simulink model "bee2_complex_corr"  (Simulink 7.0)
settings: Solver=ode45  StartTime=0.0  StopTime=10.0  RelTol=1e-3
undefined symbols (not defined in the file or in its folder): BEE2_usr
libraries: xbsIndex_r4 x279, xps_library x61, casper_library_misc x18
(part 3 of 4)

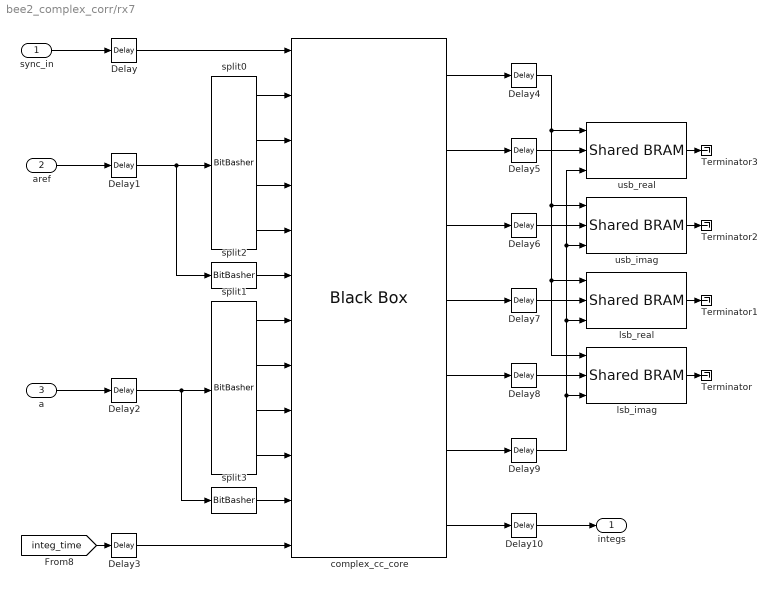
== system bee2_complex_corr/rx7 ==
  sync_in : Inport  OutDataType=sfix(16)  OutScaling=2^0
  aref : Inport  Port=2  OutDataType=sfix(16)  OutScaling=2^0
  a : Inport  Port=3  OutDataType=sfix(16)  OutScaling=2^0
  Delay{,1..10} (11 alike) : xbsIndex_r4/Delay  en=off  latency=1  dbl_ovrd=off  reg_retiming=off  block_type=delay
  Terminator{,1..3} (4 alike) : Terminator
  complex_cc_core : xbsIndex_r4/Black Box  init_code=complex_cc_core_config  sim_method=Inactive  block_type=blackbox2
      settings: infoedit="Incorporates black box HDL and simulation model into a System Generator design.<P><P>You must supply a Black Box with certain information about the HDL component you would like to bring into System Generator. This information is provided through a Matlab function.<P><P>When \"Simulation mode\" is set to \"Inactive\", you will typically want to provide a separate simulation model by using a Simulation Multiplexer.<P>When \"Simulation mode\" is set to \"External co-simulator\", you must include a ModelSim block in the design."  block_version=10.1.3
  lsb_imag : xps_library/Shared BRAM  Tag=xps:bram  SystemSampleTime=-1  arith_type="Signed  (2's comp)"  addr_width=11  data_width=32  data_bin_pt=0  init_vals=0  sample_rate=1
      link override bee2_complex_corr_0x0_func_real_data_out: arith_type="Signed  (2's comp)"
      link override bee2_complex_corr_corr00_func_real_data_out: arith_type="Signed  (2's comp)"
      link override bee2_complex_corr_corr01_func_real_data_out: arith_type="Signed  (2's comp)"
      link override bee2_complex_corr_rx7_lsb_imag_data_out: arith_type="Signed  (2's comp)"
      link override convert_din: arith_type="Signed  (2's comp)"
      link override correlator_2bit_bee2_output_corr0_data_out: arith_type=Unsigned
      link override correlator_2bit_bee2_x2_output_corr01_data_out: arith_type=Unsigned
      link override correlator_2bit_bee2_x2_output_corr0_data_out: arith_type=Unsigned
      link override correlator_2bit_ibob_output_corr0_data_out: arith_type=Unsigned
      link override cross_correlator_test_corr_out_data_out: arith_type="Signed  (2's comp)"
      link override cross_correlator_test_input_data1_data_out: arith_type=Unsigned
      link override dbe_xaui_corr_corr_func_data_out: arith_type="Signed  (2's comp)"
      link override dbe_xaui_corr_new_xaui_summer_summer_output_corr_data_out: arith_type="Signed  (2's comp)"
      link override dbe_xaui_corr_xaui_summer_summer_output_corr_data_out: arith_type="Signed  (2's comp)"
      link override mem/sim_data_in: arith_type="Signed  (2's comp)"
  lsb_real : xps_library/Shared BRAM  Tag=xps:bram  SystemSampleTime=-1  arith_type="Signed  (2's comp)"  addr_width=11  data_width=32  data_bin_pt=0  init_vals=0  sample_rate=1
      link override bee2_complex_corr_0x0_func_real_data_out: arith_type="Signed  (2's comp)"
      link override bee2_complex_corr_corr00_func_real_data_out: arith_type="Signed  (2's comp)"
      link override bee2_complex_corr_corr01_func_real_data_out: arith_type="Signed  (2's comp)"
      link override bee2_complex_corr_rx7_lsb_real_data_out: arith_type="Signed  (2's comp)"
      link override convert_din: arith_type="Signed  (2's comp)"
      link override correlator_2bit_bee2_output_corr0_data_out: arith_type=Unsigned
      link override correlator_2bit_bee2_x2_output_corr01_data_out: arith_type=Unsigned
      link override correlator_2bit_bee2_x2_output_corr0_data_out: arith_type=Unsigned
      link override correlator_2bit_ibob_output_corr0_data_out: arith_type=Unsigned
      link override cross_correlator_test_corr_out_data_out: arith_type="Signed  (2's comp)"
      link override cross_correlator_test_input_data1_data_out: arith_type=Unsigned
      link override dbe_xaui_corr_corr_func_data_out: arith_type="Signed  (2's comp)"
      link override dbe_xaui_corr_new_xaui_summer_summer_output_corr_data_out: arith_type="Signed  (2's comp)"
      link override dbe_xaui_corr_xaui_summer_summer_output_corr_data_out: arith_type="Signed  (2's comp)"
      link override mem/sim_data_in: arith_type="Signed  (2's comp)"
  split0 : xbsIndex_r4/BitBasher  bitexpr=|  display_expr=off  sr_1=1  arith_type1=Unsigned  bin_pt1=0  sr_2=2  arith_type2=Unsigned  bin_pt2=0  sr_3=3  arith_type3=Unsigned  bin_pt3=0  sr_4=4  arith_type4=Unsigned  bin_pt4=0  dbl_ovrd=off  block_type=bitbasher
      | <html><head><meta name="qrichtext" content="1" /><style type="text/css">
      | p, li { white-space: pre-wrap; }
      | </style></head><body style=" font-family:'MS Shell Dlg 2'; font-size:8.25pt; font-weight:400; font-style:normal;">
      | <p style=" margin-top:0px; margin-bottom:0px; margin-left:0px; margin-right:0px; -qt-block-indent:0; text-indent:0px; font-size:8pt;">r0={a[8:7]}<br />i0={a[6:5]}<br /><span style=" font-family:'MS Shell Dlg';">r1={a[4:3]}<br />i1={a[2:1]}</span></p></body></html>
      settings: block_version=10.1.3
  split1 : xbsIndex_r4/BitBasher  bitexpr=|  display_expr=off  sr_1=1  arith_type1=Unsigned  bin_pt1=0  sr_2=2  arith_type2=Unsigned  bin_pt2=0  sr_3=3  arith_type3=Unsigned  bin_pt3=0  sr_4=4  arith_type4=Unsigned  bin_pt4=0  dbl_ovrd=off  block_type=bitbasher
      | <html><head><meta name="qrichtext" content="1" /><style type="text/css">
      | p, li { white-space: pre-wrap; }
      | </style></head><body style=" font-family:'MS Shell Dlg 2'; font-size:8.25pt; font-weight:400; font-style:normal;">
      | <p style=" margin-top:0px; margin-bottom:0px; margin-left:0px; margin-right:0px; -qt-block-indent:0; text-indent:0px; font-size:8pt;">r0={a[8:7]}<br />i0={a[6:5]}<br /><span style=" font-family:'MS Shell Dlg';">r1={a[4:3]}<br />i1={a[2:1]}</span></p></body></html>
      settings: block_version=10.1.3
  split2 : xbsIndex_r4/BitBasher  bitexpr=|  display_expr=off  sr_1=1  arith_type1=Unsigned  bin_pt1=0  sr_2=2  arith_type2=Unsigned  bin_pt2=0  sr_3=3  arith_type3=Unsigned  bin_pt3=0  sr_4=4  arith_type4=Unsigned  bin_pt4=0  dbl_ovrd=off  block_type=bitbasher
      | <html><head><meta name="qrichtext" content="1" /><style type="text/css">
      | p, li { white-space: pre-wrap; }
      | </style></head><body style=" font-family:'MS Shell Dlg 2'; font-size:8.25pt; font-weight:400; font-style:normal;">
      | <p style=" margin-top:0px; margin-bottom:0px; margin-left:0px; margin-right:0px; -qt-block-indent:0; text-indent:0px; font-size:8pt;"><span style=" font-family:'MS Shell Dlg';">w={a[0]}</span></p></body></html>
      settings: block_version=10.1.3
  split3 : xbsIndex_r4/BitBasher  bitexpr=|  display_expr=off  sr_1=1  arith_type1=Unsigned  bin_pt1=0  sr_2=2  arith_type2=Unsigned  bin_pt2=0  sr_3=3  arith_type3=Unsigned  bin_pt3=0  sr_4=4  arith_type4=Unsigned  bin_pt4=0  dbl_ovrd=off  block_type=bitbasher
      | <html><head><meta name="qrichtext" content="1" /><style type="text/css">
      | p, li { white-space: pre-wrap; }
      | </style></head><body style=" font-family:'MS Shell Dlg 2'; font-size:8.25pt; font-weight:400; font-style:normal;">
      | <p style=" margin-top:0px; margin-bottom:0px; margin-left:0px; margin-right:0px; -qt-block-indent:0; text-indent:0px; font-size:8pt;"><span style=" font-family:'MS Shell Dlg';">w={a[0]}</span></p></body></html>
      settings: block_version=10.1.3
  usb_imag : xps_library/Shared BRAM  Tag=xps:bram  SystemSampleTime=-1  arith_type="Signed  (2's comp)"  addr_width=11  data_width=32  data_bin_pt=0  init_vals=0  sample_rate=1
      link override bee2_complex_corr_0x0_func_real_data_out: arith_type="Signed  (2's comp)"
      link override bee2_complex_corr_corr00_func_real_data_out: arith_type="Signed  (2's comp)"
      link override bee2_complex_corr_corr01_func_real_data_out: arith_type="Signed  (2's comp)"
      link override bee2_complex_corr_rx7_usb_imag_data_out: arith_type="Signed  (2's comp)"
      link override convert_din: arith_type="Signed  (2's comp)"
      link override correlator_2bit_bee2_output_corr0_data_out: arith_type=Unsigned
      link override correlator_2bit_bee2_x2_output_corr01_data_out: arith_type=Unsigned
      link override correlator_2bit_bee2_x2_output_corr0_data_out: arith_type=Unsigned
      link override correlator_2bit_ibob_output_corr0_data_out: arith_type=Unsigned
      link override cross_correlator_test_corr_out_data_out: arith_type="Signed  (2's comp)"
      link override cross_correlator_test_input_data1_data_out: arith_type=Unsigned
      link override dbe_xaui_corr_corr_func_data_out: arith_type="Signed  (2's comp)"
      link override dbe_xaui_corr_new_xaui_summer_summer_output_corr_data_out: arith_type="Signed  (2's comp)"
      link override dbe_xaui_corr_xaui_summer_summer_output_corr_data_out: arith_type="Signed  (2's comp)"
      link override mem/sim_data_in: arith_type="Signed  (2's comp)"
  usb_real : xps_library/Shared BRAM  Tag=xps:bram  SystemSampleTime=-1  arith_type="Signed  (2's comp)"  addr_width=11  data_width=32  data_bin_pt=0  init_vals=0  sample_rate=1
      link override bee2_complex_corr_0x0_func_real_data_out: arith_type="Signed  (2's comp)"
      link override bee2_complex_corr_corr00_func_real_data_out: arith_type="Signed  (2's comp)"
      link override bee2_complex_corr_corr01_func_real_data_out: arith_type="Signed  (2's comp)"
      link override bee2_complex_corr_rx7_usb_real_data_out: arith_type="Signed  (2's comp)"
      link override convert_din: arith_type="Signed  (2's comp)"
      link override correlator_2bit_bee2_output_corr0_data_out: arith_type=Unsigned
      link override correlator_2bit_bee2_x2_output_corr01_data_out: arith_type=Unsigned
      link override correlator_2bit_bee2_x2_output_corr0_data_out: arith_type=Unsigned
      link override correlator_2bit_ibob_output_corr0_data_out: arith_type=Unsigned
      link override cross_correlator_test_corr_out_data_out: arith_type="Signed  (2's comp)"
      link override cross_correlator_test_input_data1_data_out: arith_type=Unsigned
      link override dbe_xaui_corr_corr_func_data_out: arith_type="Signed  (2's comp)"
      link override dbe_xaui_corr_new_xaui_summer_summer_output_corr_data_out: arith_type="Signed  (2's comp)"
      link override dbe_xaui_corr_xaui_summer_summer_output_corr_data_out: arith_type="Signed  (2's comp)"
      link override mem/sim_data_in: arith_type="Signed  (2's comp)"
  integs : Outport  OutDataType=sfix(16)  OutScaling=2^0
  wires:
  [integ_time] -> Delay3/1
  a/1 -> Delay2/1
  aref/1 -> Delay1/1
  split0/4 -> complex_cc_core/5
  split0/3 -> complex_cc_core/4
  split0/2 -> complex_cc_core/3
  split0/1 -> complex_cc_core/2
  sync_in/1 -> Delay/1
  complex_cc_core/1 -> Delay4/1
  complex_cc_core/2 -> Delay5/1
  complex_cc_core/3 -> Delay6/1
  complex_cc_core/4 -> Delay7/1
  complex_cc_core/5 -> Delay8/1
  Delay/1 -> complex_cc_core/1
  Delay1/1 -> split0/1, split2/1
  Delay2/1 -> split1/1, split3/1
  Delay7/1 -> lsb_real/2
  Delay8/1 -> lsb_imag/2
  Delay10/1 -> integs/1
  complex_cc_core/6 -> Delay9/1
  complex_cc_core/7 -> Delay10/1
  Delay5/1 -> usb_real/2
  Delay6/1 -> usb_imag/2
  Delay3/1 -> complex_cc_core/12
  split2/1 -> complex_cc_core/6
  split1/1 -> complex_cc_core/7
  split1/2 -> complex_cc_core/8
  split1/3 -> complex_cc_core/9
  split1/4 -> complex_cc_core/10
  split3/1 -> complex_cc_core/11
  Delay4/1 -> usb_real/1, usb_imag/1, lsb_imag/1, lsb_real/1
  Delay9/1 -> usb_real/3, usb_imag/3, lsb_real/3, lsb_imag/3
  lsb_imag/1 -> Terminator/1
  lsb_real/1 -> Terminator1/1
  usb_imag/1 -> Terminator2/1
  usb_real/1 -> Terminator3/1

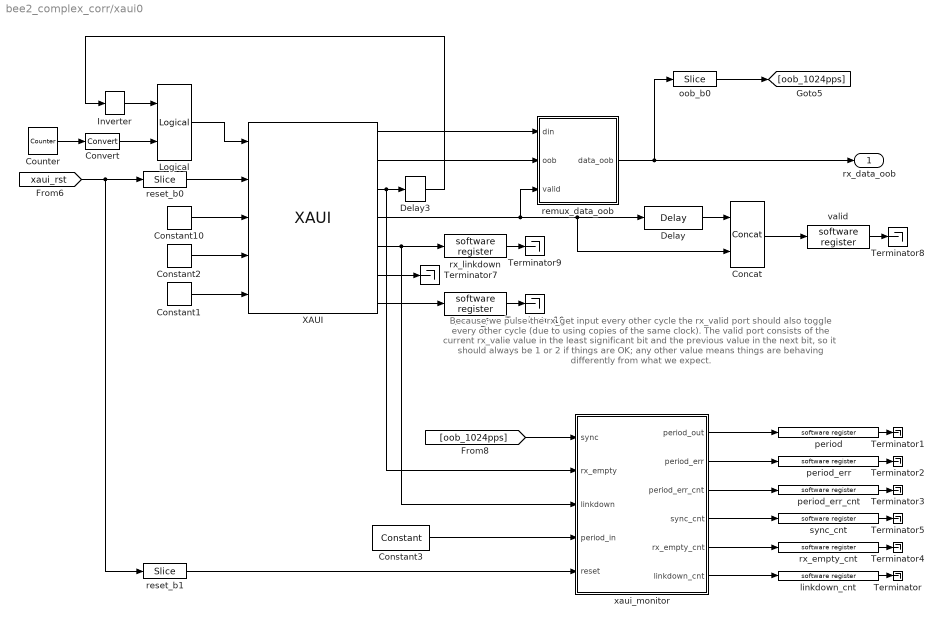
== system bee2_complex_corr/xaui0 ==
  note: Because we pulse the rx_get input every other cycle
      | the rx_valid port should also toggle every other cycle
      | (due to using copies of the same clock).  The valid port
      | consists of the current rx_valie value in the least significant
      | bit and the previous value in the next bit, so it should
      | always be 1 or 2 if things are OK; any other value means
      | things are behaving differently from what we expect.
  Concat : xbsIndex_r4/Concat  num_inputs=2  dbl_ovrd=off  block_type=concat
      settings: block_version=10.1.3
  Constant1 : xbsIndex_r4/Constant  arith_type=Boolean  const=0  n_bits=4  bin_pt=0  explicit_period=on  period=1  equ=P=C  opselect=C  inp2=PCIN>>17  opr=+  inp1=P  carry=CIN  dbl_ovrd=off  block_type=constant
      settings: block_version=11.3
  Constant10 : xbsIndex_r4/Constant  arith_type=Unsigned  const=2^4 -1  n_bits=32  bin_pt=0  explicit_period=on  period=1  equ=P=C  opselect=C  inp2=PCIN>>17  opr=+  inp1=P  carry=CIN  dbl_ovrd=off  block_type=constant
      settings: block_version=11.3
  Constant2 : xbsIndex_r4/Constant  arith_type=Unsigned  const=0  n_bits=4  bin_pt=0  explicit_period=on  period=1  equ=P=C  opselect=C  inp2=PCIN>>17  opr=+  inp1=P  carry=CIN  dbl_ovrd=off  block_type=constant
      settings: block_version=11.3
  Constant3 : xbsIndex_r4/Constant  arith_type=Unsigned  const=1e6/4  n_bits=32  bin_pt=0  explicit_period=on  period=1  equ=P=C  opselect=C  inp2=PCIN>>17  opr=+  inp1=P  carry=CIN  dbl_ovrd=off  block_type=constant
      settings: block_version=11.3
  Convert : xbsIndex_r4/Convert  arith_type=Boolean  n_bits=16  bin_pt=14  quantization=Truncate  overflow=Wrap  latency=0  dbl_ovrd=off  pipeline=off  block_type=convert
      settings: block_version=10.1.3
  Counter : xbsIndex_r4/Counter  cnt_type=Free Running  cnt_to=Inf  operation=Up  start_count=0  cnt_by_val=1  arith_type=Unsigned  n_bits=1  bin_pt=0  load_pin=off  rst=off  en=off  explicit_period=on  period=1  dbl_ovrd=off  use_behavioral_HDL=off  use_rpm=off  implementation=Fabric  block_type=counter
  Delay : xbsIndex_r4/Delay  en=off  latency=1  dbl_ovrd=off  reg_retiming=off  block_type=delay
  Delay3 : xbsIndex_r4/Delay  en=off  latency=32  dbl_ovrd=off  reg_retiming=off  block_type=delay
      settings: block_version=11.3
  Inverter : xbsIndex_r4/Inverter  en=off  latency=0  dbl_ovrd=off  block_type=inv
      settings: block_version=11.3
  Logical : xbsIndex_r4/Logical  logical_function=AND  inputs=2  en=off  latency=0  precision=Full  arith_type=Unsigned  n_bits=16  bin_pt=0  align_bp=on  dbl_ovrd=off  block_type=logical
  Terminator{,1..5,7..10} (10 alike) : Terminator
  XAUI : xps_library/XAUI  Tag=xps:xaui  SystemSampleTime=-1  demux=1  port=BEE2_usr:0  open_phy=off  show_param=off  pre_emph=3  swing=800
      link override bee2_complex_corr_xaui0_XAUI_rx_data: n_bits=64
      link override bee2_complex_corr_xaui0_XAUI_rx_outofband: n_bits=8
      link override convert_tx_data: n_bits=64
      link override convert_tx_outofband: n_bits=8
      link override dbe_xaui_corr_xaui0_XAUI_rx_data: n_bits=64
      link override dbe_xaui_corr_xaui0_XAUI_rx_outofband: n_bits=8
      link override dbe_xaui_corr_xaui1_XAUI_rx_data: n_bits=64
      link override dbe_xaui_corr_xaui1_XAUI_rx_outofband: n_bits=8
      link override dbe_xaui_corr_xaui_summer_XAUI0_rx_data: n_bits=32
      link override dbe_xaui_corr_xaui_summer_XAUI0_rx_outofband: n_bits=4
      link override dbe_xaui_xaui_summer_XAUI0_rx_data: n_bits=32
      link override dbe_xaui_xaui_summer_XAUI0_rx_outofband: n_bits=4
      link override xaui_XAUI_RECV_rx_data: n_bits=32
      link override xaui_XAUI_RECV_rx_outofband: n_bits=4
  almost_full : xps_library/software register  Tag=xps:sw_reg  SystemSampleTime=-1  io_dir=To Processor  arith_type=Unsigned  bitwidth=32  bin_pt=0  sample_period=1  gw_name=bee2_complex_corr_xaui0_almost_full_user_data_in
      link override convert: arith_type=Unsigned  n_bits=32  bin_pt=0
  linkdown_cnt : xps_library/software register  Tag=xps:sw_reg  SystemSampleTime=-1  io_dir=To Processor  arith_type=Unsigned  bitwidth=32  bin_pt=0  sample_period=1  gw_name=bee2_complex_corr_xaui0_linkdown_cnt_user_data_in
      link override convert: arith_type=Unsigned  n_bits=32  bin_pt=0
  oob_b0 : xbsIndex_r4/Slice  nbits=1  boolean_output=on  mode=Lower Bit Location + Width  bit1=0  base1=MSB of Input  bit0=0  base0=LSB of Input  dbl_ovrd=off  block_type=slice
      settings: block_version=11.3
  period : xps_library/software register  Tag=xps:sw_reg  SystemSampleTime=-1  io_dir=To Processor  arith_type=Unsigned  bitwidth=32  bin_pt=0  sample_period=1  gw_name=bee2_complex_corr_xaui0_period_user_data_in
      link override convert: arith_type=Unsigned  n_bits=32  bin_pt=0
  period_err : xps_library/software register  Tag=xps:sw_reg  SystemSampleTime=-1  io_dir=To Processor  arith_type=Unsigned  bitwidth=32  bin_pt=0  sample_period=1  gw_name=bee2_complex_corr_xaui0_period_err_user_data_in
      link override convert: arith_type=Unsigned  n_bits=32  bin_pt=0
  period_err_cnt : xps_library/software register  Tag=xps:sw_reg  SystemSampleTime=-1  io_dir=To Processor  arith_type=Unsigned  bitwidth=32  bin_pt=0  sample_period=1  gw_name=bee2_complex_corr_xaui0_period_err_cnt_user_data_in
      link override convert: arith_type=Unsigned  n_bits=32  bin_pt=0
  remux_data_oob : Subsystem
  reset_b0 : xbsIndex_r4/Slice  nbits=1  boolean_output=on  mode=Lower Bit Location + Width  bit1=0  base1=MSB of Input  bit0=0  base0=LSB of Input  dbl_ovrd=off  block_type=slice
      settings: block_version=11.3
  reset_b1 : xbsIndex_r4/Slice  nbits=1  boolean_output=on  mode=Lower Bit Location + Width  bit1=0  base1=MSB of Input  bit0=1  base0=LSB of Input  dbl_ovrd=off  block_type=slice
      settings: block_version=11.3
  rx_empty_cnt : xps_library/software register  Tag=xps:sw_reg  SystemSampleTime=-1  io_dir=To Processor  arith_type=Unsigned  bitwidth=32  bin_pt=0  sample_period=1  gw_name=bee2_complex_corr_xaui0_rx_empty_cnt_user_data_in
      link override convert: arith_type=Unsigned  n_bits=32  bin_pt=0
  rx_linkdown : xps_library/software register  Tag=xps:sw_reg  SystemSampleTime=-1  io_dir=To Processor  arith_type=Unsigned  bitwidth=32  bin_pt=0  sample_period=1  gw_name=bee2_complex_corr_xaui0_rx_linkdown_user_data_in
      link override convert: arith_type=Unsigned  n_bits=32  bin_pt=0
  sync_cnt : xps_library/software register  Tag=xps:sw_reg  SystemSampleTime=-1  io_dir=To Processor  arith_type=Unsigned  bitwidth=32  bin_pt=0  sample_period=1  gw_name=bee2_complex_corr_xaui0_sync_cnt_user_data_in
      link override convert: arith_type=Unsigned  n_bits=32  bin_pt=0
  valid : xps_library/software register  Tag=xps:sw_reg  SystemSampleTime=-1  io_dir=To Processor  arith_type=Unsigned  bitwidth=32  bin_pt=0  sample_period=1  gw_name=bee2_complex_corr_xaui0_valid_user_data_in
      link override convert: arith_type=Unsigned  n_bits=32  bin_pt=0
  xaui_monitor : Subsystem
  rx_data_oob : Outport
  wires:
  Constant2/1 -> XAUI/4
  XAUI/3 -> Delay3/1, xaui_monitor/2(rx_empty)
  Delay3/1 -> Inverter/1
  XAUI/6 -> Terminator7/1
  Constant10/1 -> XAUI/3
  XAUI/4 -> Delay/1, Concat/2, remux_data_oob/3(valid)
  XAUI/5 -> rx_linkdown/1, xaui_monitor/3(linkdown)
  valid/1 -> Terminator8/1
  rx_linkdown/1 -> Terminator9/1
  almost_full/1 -> Terminator10/1
  XAUI/7 -> almost_full/1
  Constant1/1 -> XAUI/5
  [xaui_rst] -> reset_b0/1, reset_b1/1
  Inverter/1 -> Logical/1
  Logical/1 -> XAUI/1
  Counter/1 -> Convert/1
  XAUI/1 -> remux_data_oob/1(din)
  Concat/1 -> valid/1
  Delay/1 -> Concat/1
  Convert/1 -> Logical/2
  remux_data_oob/1(data_oob) -> oob_b0/1, rx_data_oob/1
  reset_b0/1 -> XAUI/2
  reset_b1/1 -> xaui_monitor/5(reset)
  Constant3/1 -> xaui_monitor/4(period_in)
  [oob_1024pps] -> xaui_monitor/1(sync)
  oob_b0/1 -> [oob_1024pps]
  xaui_monitor/1(period_out) -> period/1
  xaui_monitor/2(period_err) -> period_err/1
  xaui_monitor/3(period_err_cnt) -> period_err_cnt/1
  xaui_monitor/4(sync_cnt) -> sync_cnt/1
  xaui_monitor/5(rx_empty_cnt) -> rx_empty_cnt/1
  xaui_monitor/6(linkdown_cnt) -> linkdown_cnt/1
  linkdown_cnt/1 -> Terminator/1
  period/1 -> Terminator1/1
  period_err/1 -> Terminator2/1
  period_err_cnt/1 -> Terminator3/1
  rx_empty_cnt/1 -> Terminator4/1
  sync_cnt/1 -> Terminator5/1
  XAUI/2 -> remux_data_oob/2(oob)

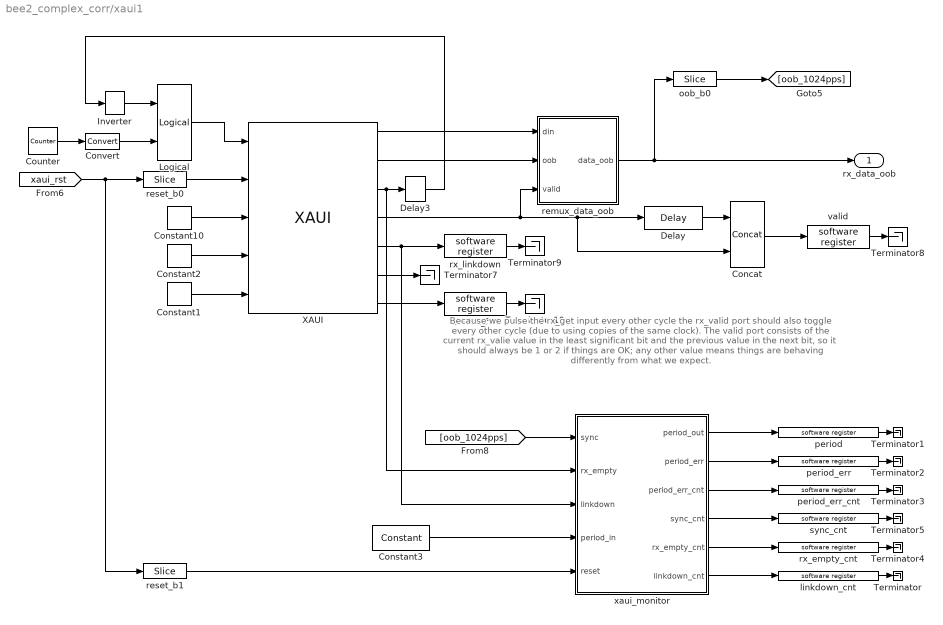
== system bee2_complex_corr/xaui1 ==
  note: Because we pulse the rx_get input every other cycle
      | the rx_valid port should also toggle every other cycle
      | (due to using copies of the same clock).  The valid port
      | consists of the current rx_valie value in the least significant
      | bit and the previous value in the next bit, so it should
      | always be 1 or 2 if things are OK; any other value means
      | things are behaving differently from what we expect.
  Concat : xbsIndex_r4/Concat  num_inputs=2  dbl_ovrd=off  block_type=concat
      settings: block_version=10.1.3
  Constant1 : xbsIndex_r4/Constant  arith_type=Boolean  const=0  n_bits=4  bin_pt=0  explicit_period=on  period=1  equ=P=C  opselect=C  inp2=PCIN>>17  opr=+  inp1=P  carry=CIN  dbl_ovrd=off  block_type=constant
      settings: block_version=11.3
  Constant10 : xbsIndex_r4/Constant  arith_type=Unsigned  const=2^4 -1  n_bits=32  bin_pt=0  explicit_period=on  period=1  equ=P=C  opselect=C  inp2=PCIN>>17  opr=+  inp1=P  carry=CIN  dbl_ovrd=off  block_type=constant
      settings: block_version=11.3
  Constant2 : xbsIndex_r4/Constant  arith_type=Unsigned  const=0  n_bits=4  bin_pt=0  explicit_period=on  period=1  equ=P=C  opselect=C  inp2=PCIN>>17  opr=+  inp1=P  carry=CIN  dbl_ovrd=off  block_type=constant
      settings: block_version=11.3
  Constant3 : xbsIndex_r4/Constant  arith_type=Unsigned  const=1e6/4  n_bits=32  bin_pt=0  explicit_period=on  period=1  equ=P=C  opselect=C  inp2=PCIN>>17  opr=+  inp1=P  carry=CIN  dbl_ovrd=off  block_type=constant
      settings: block_version=11.3
  Convert : xbsIndex_r4/Convert  arith_type=Boolean  n_bits=16  bin_pt=14  quantization=Truncate  overflow=Wrap  latency=0  dbl_ovrd=off  pipeline=off  block_type=convert
      settings: block_version=10.1.3
  Counter : xbsIndex_r4/Counter  cnt_type=Free Running  cnt_to=Inf  operation=Up  start_count=0  cnt_by_val=1  arith_type=Unsigned  n_bits=1  bin_pt=0  load_pin=off  rst=off  en=off  explicit_period=on  period=1  dbl_ovrd=off  use_behavioral_HDL=off  use_rpm=off  implementation=Fabric  block_type=counter
  Delay : xbsIndex_r4/Delay  en=off  latency=1  dbl_ovrd=off  reg_retiming=off  block_type=delay
  Delay3 : xbsIndex_r4/Delay  en=off  latency=32  dbl_ovrd=off  reg_retiming=off  block_type=delay
      settings: block_version=11.3
  Inverter : xbsIndex_r4/Inverter  en=off  latency=0  dbl_ovrd=off  block_type=inv
      settings: block_version=11.3
  Logical : xbsIndex_r4/Logical  logical_function=AND  inputs=2  en=off  latency=0  precision=Full  arith_type=Unsigned  n_bits=16  bin_pt=0  align_bp=on  dbl_ovrd=off  block_type=logical
  Terminator{,1..5,7..10} (10 alike) : Terminator
  XAUI : xps_library/XAUI  Tag=xps:xaui  SystemSampleTime=-1  demux=1  port=BEE2_usr:1  open_phy=off  show_param=off  pre_emph=3  swing=800
      link override bee2_complex_corr_xaui0_XAUI_rx_data: n_bits=64
      link override bee2_complex_corr_xaui0_XAUI_rx_outofband: n_bits=8
      link override bee2_complex_corr_xaui1_XAUI_rx_data: n_bits=64
      link override bee2_complex_corr_xaui1_XAUI_rx_outofband: n_bits=8
      link override convert_tx_data: n_bits=64
      link override convert_tx_outofband: n_bits=8
      link override dbe_xaui_corr_xaui0_XAUI_rx_data: n_bits=64
      link override dbe_xaui_corr_xaui0_XAUI_rx_outofband: n_bits=8
      link override dbe_xaui_corr_xaui1_XAUI_rx_data: n_bits=64
      link override dbe_xaui_corr_xaui1_XAUI_rx_outofband: n_bits=8
      link override dbe_xaui_corr_xaui_summer_XAUI0_rx_data: n_bits=32
      link override dbe_xaui_corr_xaui_summer_XAUI0_rx_outofband: n_bits=4
      link override dbe_xaui_xaui_summer_XAUI0_rx_data: n_bits=32
      link override dbe_xaui_xaui_summer_XAUI0_rx_outofband: n_bits=4
      link override xaui_XAUI_RECV_rx_data: n_bits=32
      link override xaui_XAUI_RECV_rx_outofband: n_bits=4
  almost_full : xps_library/software register  Tag=xps:sw_reg  SystemSampleTime=-1  io_dir=To Processor  arith_type=Unsigned  bitwidth=32  bin_pt=0  sample_period=1  gw_name=bee2_complex_corr_xaui1_almost_full_user_data_in
      link override convert: arith_type=Unsigned  n_bits=32  bin_pt=0
  linkdown_cnt : xps_library/software register  Tag=xps:sw_reg  SystemSampleTime=-1  io_dir=To Processor  arith_type=Unsigned  bitwidth=32  bin_pt=0  sample_period=1  gw_name=bee2_complex_corr_xaui1_linkdown_cnt_user_data_in
      link override convert: arith_type=Unsigned  n_bits=32  bin_pt=0
  oob_b0 : xbsIndex_r4/Slice  nbits=1  boolean_output=on  mode=Lower Bit Location + Width  bit1=0  base1=MSB of Input  bit0=0  base0=LSB of Input  dbl_ovrd=off  block_type=slice
      settings: block_version=11.3
  period : xps_library/software register  Tag=xps:sw_reg  SystemSampleTime=-1  io_dir=To Processor  arith_type=Unsigned  bitwidth=32  bin_pt=0  sample_period=1  gw_name=bee2_complex_corr_xaui1_period_user_data_in
      link override convert: arith_type=Unsigned  n_bits=32  bin_pt=0
  period_err : xps_library/software register  Tag=xps:sw_reg  SystemSampleTime=-1  io_dir=To Processor  arith_type=Unsigned  bitwidth=32  bin_pt=0  sample_period=1  gw_name=bee2_complex_corr_xaui1_period_err_user_data_in
      link override convert: arith_type=Unsigned  n_bits=32  bin_pt=0
  period_err_cnt : xps_library/software register  Tag=xps:sw_reg  SystemSampleTime=-1  io_dir=To Processor  arith_type=Unsigned  bitwidth=32  bin_pt=0  sample_period=1  gw_name=bee2_complex_corr_xaui1_period_err_cnt_user_data_in
      link override convert: arith_type=Unsigned  n_bits=32  bin_pt=0
  remux_data_oob : Subsystem
  reset_b0 : xbsIndex_r4/Slice  nbits=1  boolean_output=on  mode=Lower Bit Location + Width  bit1=0  base1=MSB of Input  bit0=0  base0=LSB of Input  dbl_ovrd=off  block_type=slice
      settings: block_version=11.3
  reset_b1 : xbsIndex_r4/Slice  nbits=1  boolean_output=on  mode=Lower Bit Location + Width  bit1=0  base1=MSB of Input  bit0=1  base0=LSB of Input  dbl_ovrd=off  block_type=slice
      settings: block_version=11.3
  rx_empty_cnt : xps_library/software register  Tag=xps:sw_reg  SystemSampleTime=-1  io_dir=To Processor  arith_type=Unsigned  bitwidth=32  bin_pt=0  sample_period=1  gw_name=bee2_complex_corr_xaui1_rx_empty_cnt_user_data_in
      link override convert: arith_type=Unsigned  n_bits=32  bin_pt=0
  rx_linkdown : xps_library/software register  Tag=xps:sw_reg  SystemSampleTime=-1  io_dir=To Processor  arith_type=Unsigned  bitwidth=32  bin_pt=0  sample_period=1  gw_name=bee2_complex_corr_xaui1_rx_linkdown_user_data_in
      link override convert: arith_type=Unsigned  n_bits=32  bin_pt=0
  sync_cnt : xps_library/software register  Tag=xps:sw_reg  SystemSampleTime=-1  io_dir=To Processor  arith_type=Unsigned  bitwidth=32  bin_pt=0  sample_period=1  gw_name=bee2_complex_corr_xaui1_sync_cnt_user_data_in
      link override convert: arith_type=Unsigned  n_bits=32  bin_pt=0
  valid : xps_library/software register  Tag=xps:sw_reg  SystemSampleTime=-1  io_dir=To Processor  arith_type=Unsigned  bitwidth=32  bin_pt=0  sample_period=1  gw_name=bee2_complex_corr_xaui1_valid_user_data_in
      link override convert: arith_type=Unsigned  n_bits=32  bin_pt=0
  xaui_monitor : Subsystem
  rx_data_oob : Outport
  wires:
  Constant2/1 -> XAUI/4
  XAUI/3 -> Delay3/1, xaui_monitor/2(rx_empty)
  Delay3/1 -> Inverter/1
  XAUI/6 -> Terminator7/1
  Constant10/1 -> XAUI/3
  XAUI/4 -> Delay/1, Concat/2, remux_data_oob/3(valid)
  XAUI/5 -> rx_linkdown/1, xaui_monitor/3(linkdown)
  valid/1 -> Terminator8/1
  rx_linkdown/1 -> Terminator9/1
  almost_full/1 -> Terminator10/1
  XAUI/7 -> almost_full/1
  Constant1/1 -> XAUI/5
  [xaui_rst] -> reset_b0/1, reset_b1/1
  Inverter/1 -> Logical/1
  Logical/1 -> XAUI/1
  Counter/1 -> Convert/1
  XAUI/1 -> remux_data_oob/1(din)
  Concat/1 -> valid/1
  Delay/1 -> Concat/1
  Convert/1 -> Logical/2
  remux_data_oob/1(data_oob) -> oob_b0/1, rx_data_oob/1
  reset_b0/1 -> XAUI/2
  reset_b1/1 -> xaui_monitor/5(reset)
  Constant3/1 -> xaui_monitor/4(period_in)
  [oob_1024pps] -> xaui_monitor/1(sync)
  oob_b0/1 -> [oob_1024pps]
  xaui_monitor/1(period_out) -> period/1
  xaui_monitor/2(period_err) -> period_err/1
  xaui_monitor/3(period_err_cnt) -> period_err_cnt/1
  xaui_monitor/4(sync_cnt) -> sync_cnt/1
  xaui_monitor/5(rx_empty_cnt) -> rx_empty_cnt/1
  xaui_monitor/6(linkdown_cnt) -> linkdown_cnt/1
  linkdown_cnt/1 -> Terminator/1
  period/1 -> Terminator1/1
  period_err/1 -> Terminator2/1
  period_err_cnt/1 -> Terminator3/1
  rx_empty_cnt/1 -> Terminator4/1
  sync_cnt/1 -> Terminator5/1
  XAUI/2 -> remux_data_oob/2(oob)

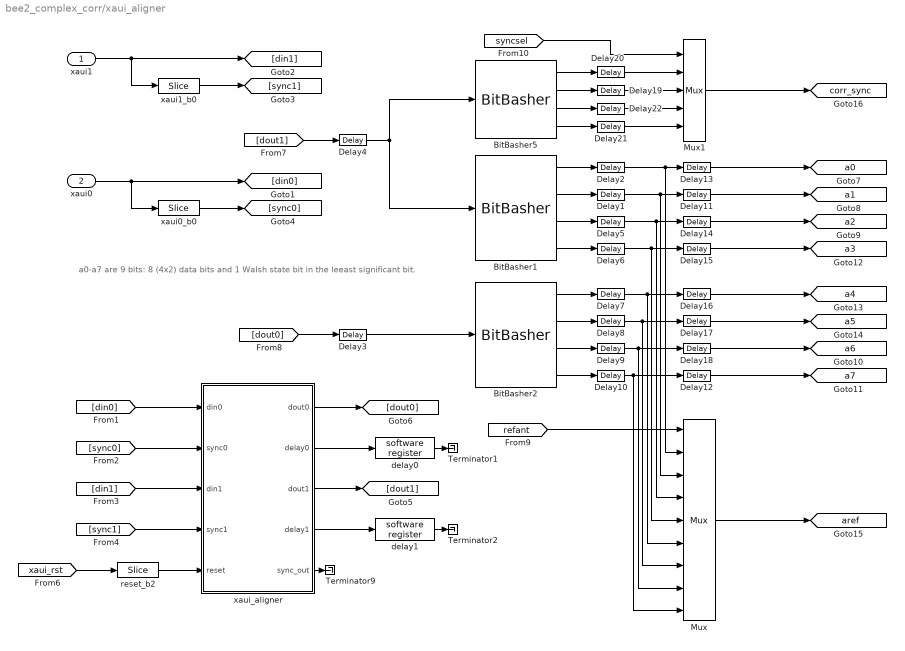
== system bee2_complex_corr/xaui_aligner ==
  note: a0-a7 are 9 bits:  8 (4x2) data bits and
      | 1 Walsh state bit in the leeast significant bit.
  xaui1 : Inport  OutDataType=sfix(16)  OutScaling=2^0
  xaui0 : Inport  Port=2  OutDataType=sfix(16)  OutScaling=2^0
  BitBasher1 : xbsIndex_r4/BitBasher  bitexpr=|  display_expr=off  sr_1=1  arith_type1=Unsigned  bin_pt1=0  sr_2=2  arith_type2=Unsigned  bin_pt2=0  sr_3=3  arith_type3=Unsigned  bin_pt3=0  sr_4=4  arith_type4=Unsigned  bin_pt4=0  dbl_ovrd=off  block_type=bitbasher
      | <html><head><meta name="qrichtext" content="1" /><style type="text/css">
      | p, li { white-space: pre-wrap; }
      | </style></head><body style=" font-family:'MS Shell Dlg 2'; font-size:8.25pt; font-weight:400; font-style:normal;">
      | <p style=" margin-top:0px; margin-bottom:0px; margin-left:0px; margin-right:0px; -qt-block-indent:0; text-indent:0px; font-size:8pt;">a0={dataoob[39:32],dataoob[4]}<br />a1={dataoob[31:24],dataoob[5]}<br />a2={dataoob[23:16],dataoob[6]}<br />a3={dataoob[15:8],dataoob[7]}<br /><br /><br /></p></body></html>
      settings: block_version=10.1.3
  BitBasher2 : xbsIndex_r4/BitBasher  bitexpr=|  display_expr=off  sr_1=1  arith_type1=Unsigned  bin_pt1=0  sr_2=2  arith_type2=Unsigned  bin_pt2=0  sr_3=3  arith_type3=Unsigned  bin_pt3=0  sr_4=4  arith_type4=Unsigned  bin_pt4=0  dbl_ovrd=off  block_type=bitbasher
      | <html><head><meta name="qrichtext" content="1" /><style type="text/css">
      | p, li { white-space: pre-wrap; }
      | </style></head><body style=" font-family:'MS Shell Dlg 2'; font-size:8.25pt; font-weight:400; font-style:normal;">
      | <p style=" margin-top:0px; margin-bottom:0px; margin-left:0px; margin-right:0px; -qt-block-indent:0; text-indent:0px; font-size:8pt;">a4={dataoob[39:32],dataoob[4]}<br />a5={dataoob[31:24],dataoob[5]}<br />a6={dataoob[23:16],dataoob[6]}<br />a7={dataoob[15:8],dataoob[7]}<br /><br /><br /></p></body></html>
      settings: block_version=10.1.3
  BitBasher5 : xbsIndex_r4/BitBasher  bitexpr=|  display_expr=off  sr_1=1  arith_type1=Unsigned  bin_pt1=0  sr_2=2  arith_type2=Unsigned  bin_pt2=0  sr_3=3  arith_type3=Unsigned  bin_pt3=0  sr_4=4  arith_type4=Unsigned  bin_pt4=0  dbl_ovrd=off  block_type=bitbasher
      | <html><head><meta name="qrichtext" content="1" /><style type="text/css">
      | p, li { white-space: pre-wrap; }
      | </style></head><body style=" font-family:'MS Shell Dlg 2'; font-size:8.25pt; font-weight:400; font-style:normal;">
      | <p style=" margin-top:0px; margin-bottom:0px; margin-left:0px; margin-right:0px; -qt-block-indent:0; text-indent:0px; font-size:8pt;">pps1024={dataoob[0]}<br />sync0={dataoob[1]}<br />sowf={dataoob[2]}<br />pps1={dataoob[3]}<br /></p></body></html>
      settings: block_version=10.1.3
  Delay{1..22} (22 alike) : xbsIndex_r4/Delay  en=off  latency=1  dbl_ovrd=off  reg_retiming=off  block_type=delay
      settings: xl_area=[0, 0, 0, 0, 0, 0, 0]  block_version=11.3
  Mux : xbsIndex_r4/Mux  inputs=8  en=off  latency=1  precision=Full  arith_type=Unsigned  n_bits=16  bin_pt=14  quantization=Truncate  overflow=Wrap  dbl_ovrd=off  block_type=mux
  Mux1 : xbsIndex_r4/Mux  inputs=4  en=off  latency=1  precision=Full  arith_type=Unsigned  n_bits=16  bin_pt=14  quantization=Truncate  overflow=Wrap  dbl_ovrd=off  block_type=mux
  Terminator1 : Terminator
  Terminator2 : Terminator
  Terminator9 : Terminator
  delay0 : xps_library/software register  Tag=xps:sw_reg  SystemSampleTime=-1  io_dir=To Processor  arith_type=Unsigned  bitwidth=32  bin_pt=0  sample_period=1  gw_name=bee2_complex_corr_xaui_aligner_delay0_user_data_in
      link override convert: arith_type=Unsigned  n_bits=32  bin_pt=0
  delay1 : xps_library/software register  Tag=xps:sw_reg  SystemSampleTime=-1  io_dir=To Processor  arith_type=Unsigned  bitwidth=32  bin_pt=0  sample_period=1  gw_name=bee2_complex_corr_xaui_aligner_delay1_user_data_in
      link override convert: arith_type=Unsigned  n_bits=32  bin_pt=0
  reset_b2 : xbsIndex_r4/Slice  nbits=1  boolean_output=on  mode=Lower Bit Location + Width  bit1=0  base1=MSB of Input  bit0=2  base0=LSB of Input  dbl_ovrd=off  block_type=slice
      settings: block_version=11.3
  xaui0_b0 : xbsIndex_r4/Slice  nbits=1  boolean_output=on  mode=Lower Bit Location + Width  bit1=0  base1=MSB of Input  bit0=0  base0=LSB of Input  dbl_ovrd=off  block_type=slice
      settings: block_version=11.3
  xaui1_b0 : xbsIndex_r4/Slice  nbits=1  boolean_output=on  mode=Lower Bit Location + Width  bit1=0  base1=MSB of Input  bit0=0  base0=LSB of Input  dbl_ovrd=off  block_type=slice
      settings: block_version=11.3
  xaui_aligner : Subsystem
  tag scope: a0=global, a1=global, a2=global, a3=global, a4=global, a5=global, a6=global, a7=global, aref=global, corr_sync=global
  wires:
  xaui1_b0/1 -> [sync1]
  xaui0_b0/1 -> [sync0]
  xaui1/1 -> [din1], xaui1_b0/1
  xaui0/1 -> [din0], xaui0_b0/1
  [din0] -> xaui_aligner/1(din0)
  [sync0] -> xaui_aligner/2(sync0)
  [din1] -> xaui_aligner/3(din1)
  [sync1] -> xaui_aligner/4(sync1)
  [xaui_rst] -> reset_b2/1
  xaui_aligner/3(dout1) -> [dout1]
  xaui_aligner/1(dout0) -> [dout0]
  xaui_aligner/2(delay0) -> delay0/1
  xaui_aligner/4(delay1) -> delay1/1
  [dout0] -> Delay3/1
  [dout1] -> Delay4/1
  delay0/1 -> Terminator1/1
  delay1/1 -> Terminator2/1
  xaui_aligner/5(sync_out) -> Terminator9/1
  Delay4/1 -> BitBasher1/1, BitBasher5/1
  Delay3/1 -> BitBasher2/1
  reset_b2/1 -> xaui_aligner/5(reset)
  BitBasher1/1 -> Delay2/1
  BitBasher1/2 -> Delay1/1
  BitBasher1/3 -> Delay5/1
  BitBasher1/4 -> Delay6/1
  BitBasher2/1 -> Delay7/1
  BitBasher2/2 -> Delay8/1
  BitBasher2/3 -> Delay9/1
  BitBasher2/4 -> Delay10/1
  BitBasher5/1 -> Delay20/1
  Delay2/1 -> Delay13/1, Mux/2
  Delay13/1 -> [a0]
  Delay1/1 -> Delay11/1, Mux/3
  Delay11/1 -> [a1]
  Delay5/1 -> Delay14/1, Mux/4
  Delay14/1 -> [a2]
  Delay6/1 -> Delay15/1, Mux/5
  Delay15/1 -> [a3]
  Delay7/1 -> Delay16/1, Mux/6
  Delay16/1 -> [a4]
  Delay8/1 -> Delay17/1, Mux/7
  Delay17/1 -> [a5]
  Delay9/1 -> Delay18/1, Mux/8
  Delay18/1 -> [a6]
  Delay10/1 -> Delay12/1, Mux/9
  Delay12/1 -> [a7]
  Delay19/1 -> Mux1/3
  [refant] -> Mux/1
  Mux/1 -> [aref]
  BitBasher5/2 -> Delay19/1
  Delay20/1 -> Mux1/2
  Mux1/1 -> [corr_sync]
  [syncsel] -> Mux1/1
  Delay22/1 -> Mux1/4
  Delay21/1 -> Mux1/5
  BitBasher5/3 -> Delay22/1
  BitBasher5/4 -> Delay21/1

== system bee2_complex_corr/xaui0/remux_data_oob ==
  note: ___     ___     ___     ___
      | valid      __/   \___/   \___/   \___/   \_
      |
      |               _______
      | oob[0]     __/       \_____________________
      |                  A       B
      |            ______ _________________________
      | wreg[3:0]  ______X_________________________
      |                    A
      |            __________ _____________________
      | wout[3:0]  __________X_____________________
      |                        A
      |                            ___
      | sync0      _______________/   \____________
      |                             B
      |                   ___
      | 1pps       ______/   \_____________________
      |                    A
      |                   ___
      | 1024pps    ______/   \_____________________
      |                    A
      |            __ _______ _______ _______ _____
      | rx[63:32]  __X_______X_______X_______X_____
      |                  0       2       4
      |            __ _______ _______ _______ _____
      | rx[31:0]   __X_______X_______X_______X_____
      |                  1       3       5
      |            ______ _______ _______ _______ _
      | first      ______X_______X_______X_______X_
      |                      0       2       4
      |            __________ _______ _______ ___ _
      | second     ______X_______X_______X_______X_
      |                      1       3       5
      |            __ ___ ___ ___ ___ ___ ___ ___ _
      | dout       __X___X___X___X___X___X___X___X_
      |                        0   1   2   3   4
  din : Inport
  oob : Inport  Port=2
  valid : Inport  Port=3
  BitBasher : xbsIndex_r4/BitBasher  bitexpr=|  display_expr=off  sr_1=1  arith_type1=Unsigned  bin_pt1=0  sr_2=2  arith_type2=Unsigned  bin_pt2=0  sr_3=3  arith_type3=Unsigned  bin_pt3=0  sr_4=4  arith_type4=Unsigned  bin_pt4=0  dbl_ovrd=off  block_type=bitbasher
      | <html><head><meta name="qrichtext" content="1" /><style type="text/css">
      | p, li { white-space: pre-wrap; }
      | </style></head><body style=" font-family:'MS Shell Dlg 2'; font-size:8.25pt; font-weight:400; font-style:normal;">
      | <p style=" margin-top:12px; margin-bottom:12px; margin-left:0px; margin-right:0px; -qt-block-indent:0; text-indent:0px; font-family:'MS Shell Dlg'; font-size:8pt;">first={din[63:32]}<br />second={din[31:0]}</p></body></html>
      settings: block_version=10.1.3
  BitBasher1 : xbsIndex_r4/BitBasher  bitexpr=|  display_expr=off  sr_1=1  arith_type1=Unsigned  bin_pt1=0  sr_2=2  arith_type2=Unsigned  bin_pt2=0  sr_3=3  arith_type3=Unsigned  bin_pt3=0  sr_4=4  arith_type4=Unsigned  bin_pt4=0  dbl_ovrd=off  block_type=bitbasher
      | <html><head><meta name="qrichtext" content="1" /><style type="text/css">
      | p, li { white-space: pre-wrap; }
      | </style></head><body style=" font-family:'MS Shell Dlg 2'; font-size:8.25pt; font-weight:400; font-style:normal;">
      | <p style=" margin-top:12px; margin-bottom:12px; margin-left:0px; margin-right:0px; -qt-block-indent:0; text-indent:0px; font-family:'MS Shell Dlg'; font-size:8pt;">pps1={oob[3]}<br />sowf={oob[2]}<br />hb={oob[1]}<br />pps1024={oob[0]}</p></body></html>
      settings: block_version=10.1.3
  BitBasher2 : xbsIndex_r4/BitBasher  bitexpr=|  display_expr=off  sr_1=1  arith_type1=Unsigned  bin_pt1=0  sr_2=2  arith_type2=Unsigned  bin_pt2=0  sr_3=3  arith_type3=Unsigned  bin_pt3=0  sr_4=4  arith_type4=Unsigned  bin_pt4=0  dbl_ovrd=off  block_type=bitbasher
      | <html><head><meta name="qrichtext" content="1" /><style type="text/css">
      | p, li { white-space: pre-wrap; }
      | </style></head><body style=" font-family:'MS Shell Dlg 2'; font-size:8.25pt; font-weight:400; font-style:normal;">
      | <p style=" margin-top:12px; margin-bottom:12px; margin-left:0px; margin-right:0px; -qt-block-indent:0; text-indent:0px; font-family:'MS Shell Dlg'; font-size:8pt;">w={oob[7:4]}<br /></p></body></html>
      settings: block_version=10.1.3
  Concat : xbsIndex_r4/Concat  num_inputs=6  dbl_ovrd=off  block_type=concat
      settings: block_version=10.1.3
  Delay1 : xbsIndex_r4/Delay  en=off  latency=1  dbl_ovrd=off  reg_retiming=off  block_type=delay
  Delay2 : xbsIndex_r4/Delay  en=off  latency=1  dbl_ovrd=off  reg_retiming=off  block_type=delay
  Inverter : xbsIndex_r4/Inverter  en=off  latency=0  dbl_ovrd=off  block_type=inv
  Mux : xbsIndex_r4/Mux  inputs=2  en=off  latency=1  precision=Full  arith_type=Unsigned  n_bits=16  bin_pt=14  quantization=Truncate  overflow=Wrap  dbl_ovrd=off  block_type=mux
  Register : xbsIndex_r4/Register  init=0  rst=off  en=on  dbl_ovrd=off  block_type=register
  Register1 : xbsIndex_r4/Register  init=0  rst=off  en=on  dbl_ovrd=off  block_type=register
  Register2 : xbsIndex_r4/Register  init=0  rst=off  en=on  dbl_ovrd=off  block_type=register
  edge_detect{,1..3} (4 alike) : casper_library_misc/edge_detect  SystemSampleTime=-1  edge=Rising  polarity=Active High  x_in=[0 0.08 0.08 0.16 0.16 0.24 0.24 0.32 0.32 0.4]  y_in="[-1 -1  1  1  1  1  1  1  1  1]"  x_out=[0.6 0.68 0.68 0.76 0.76 0.84 0.84 0.92 0.92 1]  y_out="[-1 -1  1  1 -1 -1 -1 -1 -1 -1]"
  data_oob : Outport
  wires:
  BitBasher/1 -> Register/1
  valid/1 -> Inverter/1, Register/2, Delay1/1, Register2/2
  BitBasher/2 -> Register1/1
  Inverter/1 -> Register1/2
  din/1 -> BitBasher/1
  oob/1 -> Register2/1
  Register2/1 -> BitBasher1/1, BitBasher2/1
  BitBasher1/2 -> edge_detect3/1
  BitBasher1/3 -> edge_detect1/1
  BitBasher1/4 -> edge_detect2/1
  BitBasher2/1 -> Delay2/1  "wreg"
  Delay1/1 -> Mux/1
  Register/1 -> Mux/2  "first"
  Register1/1 -> Mux/3  "second"
  Mux/1 -> Concat/1  "dout"
  Delay2/1 -> Concat/2  "wout"
  edge_detect3/1 -> Concat/4  "sowf"
  edge_detect1/1 -> Concat/5  "hb"
  edge_detect2/1 -> Concat/6  "1024pps"
  BitBasher1/1 -> edge_detect/1
  Concat/1 -> data_oob/1
  edge_detect/1 -> Concat/3  "pps1"

== system bee2_complex_corr/xaui0/xaui_monitor ==
  note: Three outputs from sync monitor have latency 5 (from sync).
      | All other outputs have latency 3 (from respective input).
  sync : Inport
  rx_empty : Inport  Port=2
  linkdown : Inport  Port=3
  period_in : Inport  Port=4
  reset : Inport  Port=5
  linkdown_counter : Subsystem
      settings: AttributesFormatString=rising
  rx_empty_counter : Subsystem
      settings: AttributesFormatString=rising
  sync_counter : Subsystem
      settings: AttributesFormatString=rising
  sync_monitor : Subsystem
  period_out : Outport
  period_err : Outport  Port=2
  period_err_cnt : Outport  Port=3
  sync_cnt : Outport  Port=4
  rx_empty_cnt : Outport  Port=5
  linkdown_cnt : Outport  Port=6
  wires:
  sync/1 -> sync_monitor/1(in), sync_counter/1(in)
  sync_monitor/1(err_count) -> period_err_cnt/1
  period_in/1 -> sync_monitor/2(expected)
  sync_monitor/2(measured) -> period_out/1
  sync_monitor/3(last_err) -> period_err/1
  sync_counter/1(count) -> sync_cnt/1
  rx_empty/1 -> rx_empty_counter/1(in)
  rx_empty_counter/1(count) -> rx_empty_cnt/1
  linkdown/1 -> linkdown_counter/1(in)
  linkdown_counter/1(count) -> linkdown_cnt/1
  reset/1 -> sync_monitor/3(reset), sync_counter/2(reset), rx_empty_counter/2(reset), linkdown_counter/2(reset)

== system bee2_complex_corr/xaui1/remux_data_oob ==
  note: ___     ___     ___     ___
      | valid      __/   \___/   \___/   \___/   \_
      |
      |               _______
      | oob[0]     __/       \_____________________
      |                  A       B
      |            ______ _________________________
      | wreg[3:0]  ______X_________________________
      |                    A
      |            __________ _____________________
      | wout[3:0]  __________X_____________________
      |                        A
      |                            ___
      | sync0      _______________/   \____________
      |                             B
      |                   ___
      | 1pps       ______/   \_____________________
      |                    A
      |                   ___
      | 1024pps    ______/   \_____________________
      |                    A
      |            __ _______ _______ _______ _____
      | rx[63:32]  __X_______X_______X_______X_____
      |                  0       2       4
      |            __ _______ _______ _______ _____
      | rx[31:0]   __X_______X_______X_______X_____
      |                  1       3       5
      |            ______ _______ _______ _______ _
      | first      ______X_______X_______X_______X_
      |                      0       2       4
      |            __________ _______ _______ ___ _
      | second     ______X_______X_______X_______X_
      |                      1       3       5
      |            __ ___ ___ ___ ___ ___ ___ ___ _
      | dout       __X___X___X___X___X___X___X___X_
      |                        0   1   2   3   4
  din : Inport
  oob : Inport  Port=2
  valid : Inport  Port=3
  BitBasher : xbsIndex_r4/BitBasher  bitexpr=|  display_expr=off  sr_1=1  arith_type1=Unsigned  bin_pt1=0  sr_2=2  arith_type2=Unsigned  bin_pt2=0  sr_3=3  arith_type3=Unsigned  bin_pt3=0  sr_4=4  arith_type4=Unsigned  bin_pt4=0  dbl_ovrd=off  block_type=bitbasher
      | <html><head><meta name="qrichtext" content="1" /><style type="text/css">
      | p, li { white-space: pre-wrap; }
      | </style></head><body style=" font-family:'MS Shell Dlg 2'; font-size:8.25pt; font-weight:400; font-style:normal;">
      | <p style=" margin-top:12px; margin-bottom:12px; margin-left:0px; margin-right:0px; -qt-block-indent:0; text-indent:0px; font-family:'MS Shell Dlg'; font-size:8pt;">first={din[63:32]}<br />second={din[31:0]}</p></body></html>
      settings: block_version=10.1.3
  BitBasher1 : xbsIndex_r4/BitBasher  bitexpr=|  display_expr=off  sr_1=1  arith_type1=Unsigned  bin_pt1=0  sr_2=2  arith_type2=Unsigned  bin_pt2=0  sr_3=3  arith_type3=Unsigned  bin_pt3=0  sr_4=4  arith_type4=Unsigned  bin_pt4=0  dbl_ovrd=off  block_type=bitbasher
      | <html><head><meta name="qrichtext" content="1" /><style type="text/css">
      | p, li { white-space: pre-wrap; }
      | </style></head><body style=" font-family:'MS Shell Dlg 2'; font-size:8.25pt; font-weight:400; font-style:normal;">
      | <p style=" margin-top:12px; margin-bottom:12px; margin-left:0px; margin-right:0px; -qt-block-indent:0; text-indent:0px; font-family:'MS Shell Dlg'; font-size:8pt;">pps1={oob[3]}<br />sowf={oob[2]}<br />hb={oob[1]}<br />pps1024={oob[0]}</p></body></html>
      settings: block_version=10.1.3
  BitBasher2 : xbsIndex_r4/BitBasher  bitexpr=|  display_expr=off  sr_1=1  arith_type1=Unsigned  bin_pt1=0  sr_2=2  arith_type2=Unsigned  bin_pt2=0  sr_3=3  arith_type3=Unsigned  bin_pt3=0  sr_4=4  arith_type4=Unsigned  bin_pt4=0  dbl_ovrd=off  block_type=bitbasher
      | <html><head><meta name="qrichtext" content="1" /><style type="text/css">
      | p, li { white-space: pre-wrap; }
      | </style></head><body style=" font-family:'MS Shell Dlg 2'; font-size:8.25pt; font-weight:400; font-style:normal;">
      | <p style=" margin-top:12px; margin-bottom:12px; margin-left:0px; margin-right:0px; -qt-block-indent:0; text-indent:0px; font-family:'MS Shell Dlg'; font-size:8pt;">w={oob[7:4]}<br /></p></body></html>
      settings: block_version=10.1.3
  Concat : xbsIndex_r4/Concat  num_inputs=6  dbl_ovrd=off  block_type=concat
      settings: block_version=10.1.3
  Delay1 : xbsIndex_r4/Delay  en=off  latency=1  dbl_ovrd=off  reg_retiming=off  block_type=delay
  Delay2 : xbsIndex_r4/Delay  en=off  latency=1  dbl_ovrd=off  reg_retiming=off  block_type=delay
  Inverter : xbsIndex_r4/Inverter  en=off  latency=0  dbl_ovrd=off  block_type=inv
  Mux : xbsIndex_r4/Mux  inputs=2  en=off  latency=1  precision=Full  arith_type=Unsigned  n_bits=16  bin_pt=14  quantization=Truncate  overflow=Wrap  dbl_ovrd=off  block_type=mux
  Register : xbsIndex_r4/Register  init=0  rst=off  en=on  dbl_ovrd=off  block_type=register
  Register1 : xbsIndex_r4/Register  init=0  rst=off  en=on  dbl_ovrd=off  block_type=register
  Register2 : xbsIndex_r4/Register  init=0  rst=off  en=on  dbl_ovrd=off  block_type=register
  edge_detect{,1..3} (4 alike) : casper_library_misc/edge_detect  SystemSampleTime=-1  edge=Rising  polarity=Active High  x_in=[0 0.08 0.08 0.16 0.16 0.24 0.24 0.32 0.32 0.4]  y_in="[-1 -1  1  1  1  1  1  1  1  1]"  x_out=[0.6 0.68 0.68 0.76 0.76 0.84 0.84 0.92 0.92 1]  y_out="[-1 -1  1  1 -1 -1 -1 -1 -1 -1]"
  data_oob : Outport
  wires:
  BitBasher/1 -> Register/1
  valid/1 -> Inverter/1, Register/2, Delay1/1, Register2/2
  BitBasher/2 -> Register1/1
  Inverter/1 -> Register1/2
  din/1 -> BitBasher/1
  oob/1 -> Register2/1
  Register2/1 -> BitBasher1/1, BitBasher2/1
  BitBasher1/2 -> edge_detect3/1
  BitBasher1/3 -> edge_detect1/1
  BitBasher1/4 -> edge_detect2/1
  BitBasher2/1 -> Delay2/1  "wreg"
  Delay1/1 -> Mux/1
  Register/1 -> Mux/2  "first"
  Register1/1 -> Mux/3  "second"
  Mux/1 -> Concat/1  "dout"
  Delay2/1 -> Concat/2  "wout"
  edge_detect3/1 -> Concat/4  "sowf"
  edge_detect1/1 -> Concat/5  "hb"
  edge_detect2/1 -> Concat/6  "1024pps"
  BitBasher1/1 -> edge_detect/1
  Concat/1 -> data_oob/1
  edge_detect/1 -> Concat/3  "pps1"

== system bee2_complex_corr/xaui1/xaui_monitor ==
  note: Three outputs from sync monitor have latency 5 (from sync).
      | All other outputs have latency 3 (from respective input).
  sync : Inport
  rx_empty : Inport  Port=2
  linkdown : Inport  Port=3
  period_in : Inport  Port=4
  reset : Inport  Port=5
  linkdown_counter : Subsystem
      settings: AttributesFormatString=rising
  rx_empty_counter : Subsystem
      settings: AttributesFormatString=rising
  sync_counter : Subsystem
      settings: AttributesFormatString=rising
  sync_monitor : Subsystem
  period_out : Outport
  period_err : Outport  Port=2
  period_err_cnt : Outport  Port=3
  sync_cnt : Outport  Port=4
  rx_empty_cnt : Outport  Port=5
  linkdown_cnt : Outport  Port=6
  wires:
  sync/1 -> sync_monitor/1(in), sync_counter/1(in)
  sync_monitor/1(err_count) -> period_err_cnt/1
  period_in/1 -> sync_monitor/2(expected)
  sync_monitor/2(measured) -> period_out/1
  sync_monitor/3(last_err) -> period_err/1
  sync_counter/1(count) -> sync_cnt/1
  rx_empty/1 -> rx_empty_counter/1(in)
  rx_empty_counter/1(count) -> rx_empty_cnt/1
  linkdown/1 -> linkdown_counter/1(in)
  linkdown_counter/1(count) -> linkdown_cnt/1
  reset/1 -> sync_monitor/3(reset), sync_counter/2(reset), rx_empty_counter/2(reset), linkdown_counter/2(reset)

== system bee2_complex_corr/xaui_aligner/xaui_aligner ==
  din0 : Inport
  sync0 : Inport  Port=2
  din1 : Inport  Port=3
  sync1 : Inport  Port=4
  reset : Inport  Port=5
  Delay20 : xbsIndex_r4/Delay  en=off  latency=1  dbl_ovrd=off  reg_retiming=off  block_type=delay
      settings: xl_area=[0, 0, 0, 0, 0, 0, 0]  block_version=11.3
  realign : Subsystem
  dout0 : Outport
  delay0 : Outport  Port=2
  dout1 : Outport  Port=3
  delay1 : Outport  Port=4
  sync_out : Outport  Port=5
  wires:
  Delay20/1 -> realign/5(sync_ref)  "sync_in"
  realign/1(dout0) -> dout0/1  "dout0"
  din0/1 -> realign/1(din0)
  sync0/1 -> realign/2(sync0)
  realign/2(delay0) -> delay0/1  "delay0"
  din1/1 -> realign/3(din1)
  realign/3(dout1) -> dout1/1  "dout1"
  sync1/1 -> realign/4(sync1), Delay20/1
  realign/4(delay1) -> delay1/1  "delay1"
  reset/1 -> realign/6(reset)
  realign/5(sync_out) -> sync_out/1  "sync_out"
